simulink model "IP_LinearSys_LQR"  (R2015a)
settings: Solver=ode5  StartTime=0.0  StopTime=20  FixedStep=0.01  RelTol=1e-3
model workspace (MAT data in the model file):
  A = [0  0  1  0; 0  0  0  1; 0  0.252647937474  -2.0942342122  -0.00013290604508; 0  15.0472557056  -3.13162876156  -0.00791564445427]
  B = [0; 0; 5.7783045915; 8.64063090286]
  C = [1  0  0  0; 0  1  0  0]
  Cfs = [1  0  0  0; 0  1  0  0; 0  0  1  0; 0  0  0  1]
  D = [0; 0]
  Dfs = [0; 0; 0; 0]
settings Model: Creator=Fares  LastModifiedBy=Fares

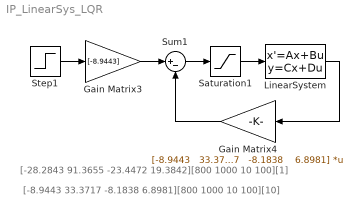
== system IP_LinearSys_LQR ==
  note: [-8.9443 33.3717 -8.1838 6.8981][800 1000 10 100][10]
  note: [-28.2843 91.3655 -23.4472 19.3842][800 1000 10 100][1]
  Gain Matrix3 : Gain  Gain=[-8.9443]
  Gain Matrix4 : Gain  Gain="[-8.9443   33.3717   -8.1838    6.8981]"  Multiplication=Matrix(K*u) (u vector)
  LinearSystem : StateSpace  A=A  B=B  C=C  D=D  X0=[0; 0; 0; 0]  mask(SS MASK){}
      mask init:
      | mc = 1.12;
      | mpw = 0.095;
      | mps = 0.025;
      | l = 0.033245968;
      | fc = 2.53165; % FS = 2.53165; FC = 2.28133
      | fp = 0.000107443;
      | J = 0.013935418;
      | g = 9.81;
      | vf = 9.4/2.5; %Voltage to Motor Force ratio
      | mp = mpw + mps;
      | a = l^2 + J/(mc + mp);
      | mu = (mc + mp)*l;
      | 
      | % theta 0 in upward position
      | % theta pi in downward position
      | s = 1; % 1 when upward  -1 when downward
      | 
      | A = [0          0              1               0;
      |      0          0              0               1;
      |      0      (l*mu*g)/J    -(a*fc)/J    -(l*fp)/J;
      |      0      s*(mu*g)/J    -s*(l*fc)/J    -(fp)/J];
      |  
      | B = [         0;
      |               0;
      |        (vf*a)/J;
      |       (s*vf*l)/J];
      |   
      | C = [1 0 0 0;
      |      0 1 0 0;
      |      0 0 1 0;
      |      0 0 0 1];
      |  
      | D = [0;
      |      0;
      |      0;
      |      0];
  Saturation1 : Saturate  UpperLimit=2.5  LowerLimit=-2.5
  Step1 : Step  Time=10  Before=-0.2  After=0.2  SampleTime=0
  Sum1 : Sum  Inputs=|+-
  wires:
  Sum1/1 -> Saturation1/1
  Gain Matrix4/1 -> Sum1/2
  Gain Matrix3/1 -> Sum1/1
  Step1/1 -> Gain Matrix3/1
  Saturation1/1 -> LinearSystem/1
  LinearSystem/1 -> Gain Matrix4/1
